simulink model "Firsts_OPTION"  (R2023a)
settings: Solver=FixedStepAuto  StartTime=0.0  StopTime=inf  FixedStep=0.01  RelTol=1e-3  EnableMultiTasking=on
libraries: arduinolib x35, dspfdesign x10, slpidlib x5
settings Model: ExtModeTrigDuration=2  Creator=PHUC  LastModifiedBy=PHUC
settings SolverCC: AutoInsertRateTranBlk=on
settings OptimizationCC: EnhancedBackFolding=on  PassReuseOutputArgsAs=Individual arguments  ZeroExternalMemoryAtStartup=off  ZeroInternalMemoryAtStartup=off  MaxStackSize=64  OptimizeBlockOrder=speed  DifferentSizesBufferReuse=on  OptimizationCustomize=off  EfficientTunableParamExpr=on
settings DebuggingCC: ParameterTunabilityLossMsg=error
settings HardwareCC: ProdBitPerInt=16  ProdBitPerPointer=16  ProdBitPerSizeT=16  ProdBitPerPtrDiffT=16  ProdLargestAtomicFloat=None  ProdWordSize=8  ProdHWDeviceType=Atmel->AVR
settings SFSimCC: MATLABDynamicMemAlloc=off
settings RTWCC: Description=Embedded Coder  SystemTargetFile=ert.tlc  HardwareBoard=Arduino Mega 2560  TemplateMakefile=ert_default_tmf  Toolchain=Arduino AVR  BuildConfiguration=Faster Runs
settings CodeAppCC: ForceParamTrailComments=on  IgnoreCustomStorageClasses=off  OperatorAnnotations=on  SimulinkDataObjDesc=on  SFDataObjDesc=on  InsertBlockDesc=on
settings ERTTargetCC: SupportContinuousTime=on  SupportVariableSizeSignals=on  ExtModeTransport=3  ExtModeStaticAlloc=on  ExtModeAutomaticAllocSize=off  ExtModeStaticAllocSize=2048  ExtModeMexFile=ext_xcp  ExtModeIntrfLevel=Level2 - Open

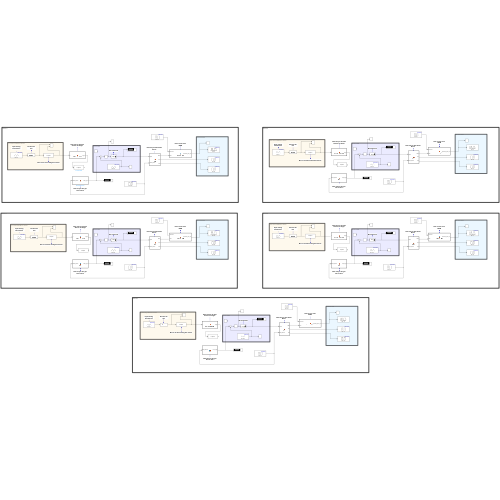
[thumbnail: Simulink's stored preview of the top-level diagram]
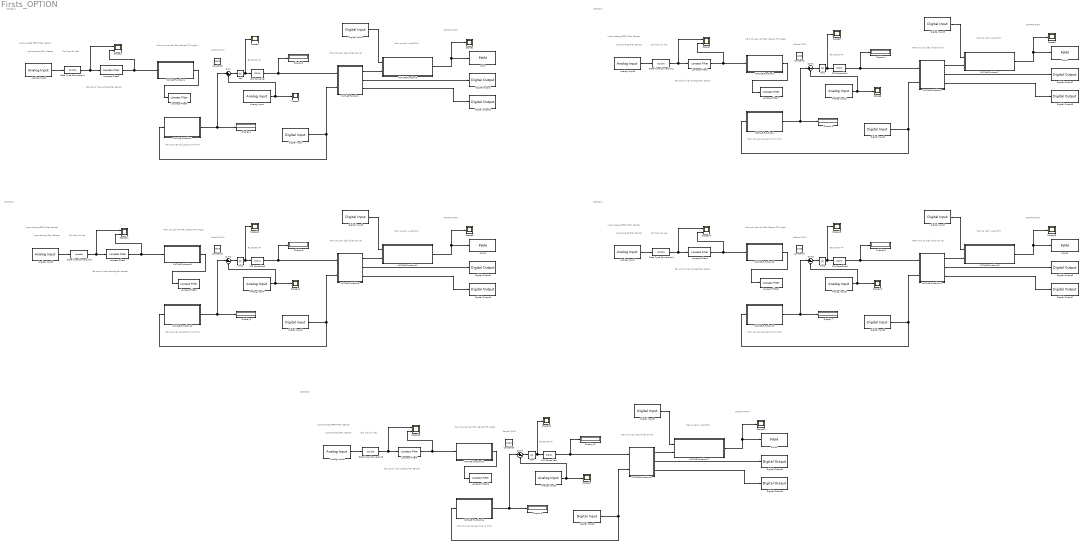
== system Firsts_OPTION ==
  note: MOTOR 1
  note: OUTPUT PWM
  note: Bo Control PI
  note: Control PWM
  note: Ham chuyen doi Flex Sensor TO Angle
  note: Doi kieu du lieu
  note: Bo Loc tin hieu analog flex sensor
  note: Input Analog FROM Flex Sensor
  note: Input analog Flex Sensor
  note: Ham chuyen dieu khien Driver
  note: Ham chuyen doi goc Hut va Thoi
  note: Ham ra lenh xuat PWM
  note: Ham ra lenh xuat PWM
  note: Doi kieu du lieu
  note: Ham chuyen doi Flex Sensor TO Angle
  note: Input analog Flex Sensor
  note: OUTPUT PWM
  note: Input Analog FROM Flex Sensor
  note: Control PWM
  note: Bo Control PI
  note: Bo Loc tin hieu analog flex sensor
  note: Ham chuyen dieu khien Driver
  note: Ham chuyen doi goc Hut va Thoi
  note: Ham ra lenh xuat PWM
  note: Control PWM
  note: Ham chuyen doi goc Hut va Thoi
  note: Input Analog FROM Flex Sensor
  note: Bo Control PI
  note: Ham chuyen dieu khien Driver
  note: Input analog Flex Sensor
  note: Bo Loc tin hieu analog flex sensor
  note: Ham chuyen doi Flex Sensor TO Angle
  note: Doi kieu du lieu
  note: OUTPUT PWM
  note: Control PWM
  note: Doi kieu du lieu
  note: Ham chuyen dieu khien Driver
  note: Ham chuyen doi Flex Sensor TO Angle
  note: OUTPUT PWM
  note: Bo Loc tin hieu analog flex sensor
  note: Bo Control PI
  note: Ham ra lenh xuat PWM
  note: Input Analog FROM Flex Sensor
  note: Input analog Flex Sensor
  note: Ham chuyen doi goc Hut va Thoi
  note: Input analog Flex Sensor
  note: Ham chuyen doi Flex Sensor TO Angle
  note: Bo Loc tin hieu analog flex sensor
  note: OUTPUT PWM
  note: Input Analog FROM Flex Sensor
  note: Ham chuyen doi goc Hut va Thoi
  note: Ham chuyen dieu khien Driver
  note: Bo Control PI
  note: Doi kieu du lieu
  note: Ham ra lenh xuat PWM
  note: Control PWM
  note: MOTOR 2
  note: MOTOR 5
  note: MOTOR 4
  note: MOTOR 3
  Abs{,1..4} (5 alike) : Abs  SaturateOnIntegerOverflow=off
  Analog Input : arduinolib/Analog Input  pinNumber=8  ReadResultsOnly=off  ConversionTriggerSource=Software  ExternalTriggerType=uint32( 0 )  OutputDataType=uint16  EnableConversionCompleteNotify=off  EnableOuputStatus=off  SampleTime=-1  blockPlatform=arduino
  Analog Input1 : arduinolib/Analog Input  pinNumber=0  ReadResultsOnly=off  ConversionTriggerSource=Software  ExternalTriggerType=uint32( 0 )  OutputDataType=uint16  EnableConversionCompleteNotify=off  EnableOuputStatus=off  SampleTime=-1  blockPlatform=arduino
  Analog Input2 : arduinolib/Analog Input  pinNumber=9  ReadResultsOnly=off  ConversionTriggerSource=Software  ExternalTriggerType=uint32( 0 )  OutputDataType=uint16  EnableConversionCompleteNotify=off  EnableOuputStatus=off  SampleTime=-1  blockPlatform=arduino
  Analog Input3 : arduinolib/Analog Input  pinNumber=1  ReadResultsOnly=off  ConversionTriggerSource=Software  ExternalTriggerType=uint32( 0 )  OutputDataType=uint16  EnableConversionCompleteNotify=off  EnableOuputStatus=off  SampleTime=-1  blockPlatform=arduino
  Analog Input4 : arduinolib/Analog Input  pinNumber=10  ReadResultsOnly=off  ConversionTriggerSource=Software  ExternalTriggerType=uint32( 0 )  OutputDataType=uint16  EnableConversionCompleteNotify=off  EnableOuputStatus=off  SampleTime=-1  blockPlatform=arduino
  Analog Input5 : arduinolib/Analog Input  pinNumber=2  ReadResultsOnly=off  ConversionTriggerSource=Software  ExternalTriggerType=uint32( 0 )  OutputDataType=uint16  EnableConversionCompleteNotify=off  EnableOuputStatus=off  SampleTime=-1  blockPlatform=arduino
  Analog Input6 : arduinolib/Analog Input  pinNumber=11  ReadResultsOnly=off  ConversionTriggerSource=Software  ExternalTriggerType=uint32( 0 )  OutputDataType=uint16  EnableConversionCompleteNotify=off  EnableOuputStatus=off  SampleTime=-1  blockPlatform=arduino
  Analog Input7 : arduinolib/Analog Input  pinNumber=3  ReadResultsOnly=off  ConversionTriggerSource=Software  ExternalTriggerType=uint32( 0 )  OutputDataType=uint16  EnableConversionCompleteNotify=off  EnableOuputStatus=off  SampleTime=-1  blockPlatform=arduino
  Analog Input8 : arduinolib/Analog Input  pinNumber=12  ReadResultsOnly=off  ConversionTriggerSource=Software  ExternalTriggerType=uint32( 0 )  OutputDataType=uint16  EnableConversionCompleteNotify=off  EnableOuputStatus=off  SampleTime=-1  blockPlatform=arduino
  Analog Input9 : arduinolib/Analog Input  pinNumber=4  ReadResultsOnly=off  ConversionTriggerSource=Software  ExternalTriggerType=uint32( 0 )  OutputDataType=uint16  EnableConversionCompleteNotify=off  EnableOuputStatus=off  SampleTime=-1  blockPlatform=arduino
  Constant{1..5} (5 alike) : Constant  Value=1023
  Data Type Conversion{1..5} (5 alike) : DataTypeConversion  OutDataTypeStr=double  SaturateOnIntegerOverflow=off  RndMeth=Floor
  Digital Input : arduinolib/Digital Input  pinNumber=34  mode=Default  Direction=input  SampleTime=0.1  blockPlatform=arduino
  Digital Input1 : arduinolib/Digital Input  pinNumber=24  mode=Default  Direction=input  SampleTime=0.1  blockPlatform=arduino
  Digital Input2 : arduinolib/Digital Input  pinNumber=36  mode=Default  Direction=input  SampleTime=0.1  blockPlatform=arduino
  Digital Input3 : arduinolib/Digital Input  pinNumber=26  mode=Default  Direction=input  SampleTime=0.1  blockPlatform=arduino
  Digital Input4 : arduinolib/Digital Input  pinNumber=38  mode=Default  Direction=input  SampleTime=0.1  blockPlatform=arduino
  Digital Input5 : arduinolib/Digital Input  pinNumber=28  mode=Default  Direction=input  SampleTime=0.1  blockPlatform=arduino
  Digital Input6 : arduinolib/Digital Input  pinNumber=40  mode=Default  Direction=input  SampleTime=0.1  blockPlatform=arduino
  Digital Input7 : arduinolib/Digital Input  pinNumber=30  mode=Default  Direction=input  SampleTime=0.1  blockPlatform=arduino
  Digital Input8 : arduinolib/Digital Input  pinNumber=42  mode=Default  Direction=input  SampleTime=0.1  blockPlatform=arduino
  Digital Input9 : arduinolib/Digital Input  pinNumber=32  mode=Default  Direction=input  SampleTime=0.1  blockPlatform=arduino
  Digital Output : arduinolib/Digital Output  pinNumber=25  Direction=output  blockPlatform=arduino
  Digital Output1 : arduinolib/Digital Output  pinNumber=27  Direction=output  blockPlatform=arduino
  Digital Output2 : arduinolib/Digital Output  pinNumber=29  Direction=output  blockPlatform=arduino
  Digital Output3 : arduinolib/Digital Output  pinNumber=31  Direction=output  blockPlatform=arduino
  Digital Output4 : arduinolib/Digital Output  pinNumber=33  Direction=output  blockPlatform=arduino
  Digital Output5 : arduinolib/Digital Output  pinNumber=35  Direction=output  blockPlatform=arduino
  Digital Output6 : arduinolib/Digital Output  pinNumber=37  Direction=output  blockPlatform=arduino
  Digital Output7 : arduinolib/Digital Output  pinNumber=39  Direction=output  blockPlatform=arduino
  Digital Output8 : arduinolib/Digital Output  pinNumber=41  Direction=output  blockPlatform=arduino
  Digital Output9 : arduinolib/Digital Output  pinNumber=43  Direction=output  blockPlatform=arduino
  Display{1..10} (10 alike) : Display
  Lowpass Filter{1..5} (5 alike) : dspfdesign/Lowpass Filter  FilterType=FIR  DesignForMinimumOrder=off  FilterOrder=200  PassbandFrequency=0.1e3  StopbandFrequency=12e3  PassbandRipple=0.01  StopbandAttenuation=50  SampleRateMode=Specify on dialog  SampleRate=44100  SimulateUsing=Interpreted execution  roundingMode=Floor  coeffsDataTypeStr=fixdt(1,16)
  Lowpass Filter{6..10} (5 alike) : dspfdesign/Lowpass Filter  FilterType=FIR  DesignForMinimumOrder=off  FilterOrder=30  PassbandFrequency=0.01e2  StopbandFrequency=12e3  PassbandRipple=0.001  StopbandAttenuation=50  SampleRateMode=Specify on dialog  SampleRate=44100  SimulateUsing=Interpreted execution  roundingMode=Floor  coeffsDataTypeStr=fixdt(1,16)
  MATLAB Function : MATLAB Function  TreatAsAtomicUnit=on
  MATLAB Function1 : MATLAB Function  TreatAsAtomicUnit=on
  MATLAB Function10 : MATLAB Function  TreatAsAtomicUnit=on
  MATLAB Function11 : MATLAB Function  TreatAsAtomicUnit=on
  MATLAB Function12 : MATLAB Function  TreatAsAtomicUnit=on
  MATLAB Function13 : MATLAB Function  TreatAsAtomicUnit=on
  MATLAB Function14 : MATLAB Function  TreatAsAtomicUnit=on
  MATLAB Function15 : MATLAB Function  TreatAsAtomicUnit=on
  MATLAB Function16 : MATLAB Function  TreatAsAtomicUnit=on
  MATLAB Function17 : MATLAB Function  TreatAsAtomicUnit=on
  MATLAB Function18 : MATLAB Function  TreatAsAtomicUnit=on
  MATLAB Function19 : MATLAB Function  TreatAsAtomicUnit=on
  MATLAB Function2 : MATLAB Function  TreatAsAtomicUnit=on
  MATLAB Function3 : MATLAB Function  TreatAsAtomicUnit=on
  MATLAB Function4 : MATLAB Function  TreatAsAtomicUnit=on
  MATLAB Function5 : MATLAB Function  TreatAsAtomicUnit=on
  MATLAB Function6 : MATLAB Function  TreatAsAtomicUnit=on
  MATLAB Function7 : MATLAB Function  TreatAsAtomicUnit=on
  MATLAB Function8 : MATLAB Function  TreatAsAtomicUnit=on
  MATLAB Function9 : MATLAB Function  TreatAsAtomicUnit=on
  PID Controller{,1..4} (5 alike) : slpidlib/PID Controller  Controller=PID  Form=Parallel  TimeDomain=Discrete-time  UseExternalTs=off  SampleTime=0.01  IntegratorMethod=Forward Euler  FilterMethod=Forward Euler  ControllerParametersSource=internal  P=7  I=0.8  UseKiTs=off  D=0  N=100  UseFilter=on  TunerSelectOption=Transfer Function Based (PID Tuner App)  InitialConditionSource=internal  InitialConditionForIntegrator=0  InitialConditionForFilter=0  DifferentiatorICPrevScaledInput=0  ExternalReset=none  TrackingMode=off  Kt=1  LimitOutput=on  SatLimitsSource=internal  UpperSaturationLimit=160  LowerSaturationLimit=0  LinearizeAsGain=on  AntiWindupMode=back-calculation  Kb=1  LimitIntegrator=off  UpperIntegratorSaturationLimit=inf  LowerIntegratorSaturationLimit=-inf  POutMin=[]  POutMax=[]  IOutMin=[]  IOutMax=[]  DOutMin=[]  DOutMax=[]  NOutMin=[]  NOutMax=[]  SumOutMin=[]  SumOutMax=[]  SaturationOutMin=[]  SaturationOutMax=[]  PParamMin=[]  PParamMax=[]  IParamMin=[]  IParamMax=[]  DParamMin=[]  DParamMax=[]  NParamMin=[]  NParamMax=[]  KbParamMin=[]  KbParamMax=[]  KtParamMin=[]  KtParamMax=[]  KbOutMin=[]  KbOutMax=[]  KtOutMin=[]  KtOutMax=[]  IntegratorOutMin=[]  IntegratorOutMax=[]  FilterOutMin=[]  FilterOutMax=[]  SumI1OutMin=[]  SumI1OutMax=[]  SumI2OutMin=[]  SumI2OutMax=[]  SumI3OutMin=[]  SumI3OutMax=[]  SumI4OutMin=[]  SumI4OutMax=[]  SumDOutMin=[]  SumDOutMax=[]  DifferentiatorOutMin=[]  DifferentiatorOutMax=[]  FilterDiffOutCoefMin=[]  FilterDiffOutCoefMax=[]  ReciprocalOutMin=[]  ReciprocalOutMax=[]  SumDenOutMin=[]  SumDenOutMax=[]  SumNumOutMin=[]  SumNumOutMax=[]  DivideOutMin=[]  DivideOutMax=[]  UdiffTsProdOutMin=[]  UdiffTsProdOutMax=[]  NTsProdOutMin=[]  NTsProdOutMax=[]  UintegralTsProdOutMin=[]  UintegralTsProdOutMax=[]  UngainTsProdOutMin=[]  UngainTsProdOutMax=[]  ClampingZeroOutDataTypeStr=Inherit: Inherit via back propagation  ClampingZeroOutMin=[]  ClampingZeroOutMax=[]  FilterDenConstantOutDataTypeStr=Inherit: Inherit via back propagation  FilterDenConstantOutMin=[]  FilterDenConstantOutMax=[]  PCopyOutDataTypeStr=Inherit: Inherit via back propagation  PCopyOutMin=[]  PCopyOutMax=[]  NCopyOutDataTypeStr=Inherit: Inherit via back propagation  NCopyOutMin=[]  NCopyOutMax=[]  IntegratorContinuousStateAttributes=''  IntegratorStateMustResolveToSignalObject=off  IntegratorRTWStateStorageClass=Auto  FilterContinuousStateAttributes=''  FilterStateMustResolveToSignalObject=off  FilterRTWStateStorageClass=Auto  ParallelPVariant=InternalParameters  IdealPVariant=Disabled  IVariant=InternalParameters  DVariant=InternalParameters  IntegratorVariant=Discrete  SatVariant=Enabled  AWVariant=BackCalculation  PCopyVariant=Disabled  TRVariant=Disabled  FdbkBlocksVariant=Forward  IdealPFdbkVariant=Disabled  SatFdbkVariant=Disabled  DerivativeFilterVariant=ForwardEulerFilter  NVariant=InternalParameters  NCopyVariant=Disabled  FilterICVariant=InternalICsFilter  IntegratorICVariant=InternalICs  ExternalResetVariant=Disabled  TRSumVariant=Passthrough  SumFdbkVariant=Disabled  SumVariant=Sum_PID  TsampFilterVariant=InternalTs  TsampNgainVariant=Passthrough  TsampIntegralVariant=Disabled_SignalSpec  ExternalSaturationOutDataTypeStr=Inherit: Same as second input
  PWM : arduinolib/PWM  pinNumber=8  frequencyType=Default  desiredFrequency=490.2  achievableFrequency=490.2
  PWM1 : arduinolib/PWM  pinNumber=9  frequencyType=Default  desiredFrequency=490.2  achievableFrequency=490.2
  PWM2 : arduinolib/PWM  pinNumber=10  frequencyType=Default  desiredFrequency=490.2  achievableFrequency=490.2
  PWM3 : arduinolib/PWM  pinNumber=11  frequencyType=Default  desiredFrequency=490.2  achievableFrequency=490.2
  PWM4 : arduinolib/PWM  pinNumber=12  frequencyType=Default  desiredFrequency=490.2  achievableFrequency=490.2
  Scope{1..2,4..6,8..10,12..13,15..17,19..20} (15 alike) : Scope
  Scope{3,7,11,14,18} (5 alike) : Scope  NumInputPorts=2
  Sum{,1..4} (5 alike) : Sum  Inputs=|+-
  wires:
  MATLAB Function/2(IN1) -> Digital Output/1
  MATLAB Function/3(IN2) -> Digital Output1/1
  PID Controller/1 -> Display2/1, MATLAB Function/1(speed)
  Digital Input/1 -> MATLAB Function/2(Blend_Stretch), MATLAB Function2/1(Blend_Stretch)
  Analog Input/1 -> Scope2/1, Sum/2
  Analog Input1/1 -> Data Type Conversion1/1
  Data Type Conversion1/1 -> Lowpass Filter3/1, Scope3/1
  Lowpass Filter3/1 -> Scope3/2, MATLAB Function1/1(u)
  MATLAB Function2/1(Limit_angle) -> Sum/1, Display1/1
  Sum/1 -> Abs/1
  Abs/1 -> Scope4/1, PID Controller/1
  Digital Input1/1 -> MATLAB Function3/1(command)
  MATLAB Function/1(ENA) -> MATLAB Function3/2(pwm)
  MATLAB Function3/1(command_pwm_out) -> Scope1/1, PWM/1
  MATLAB Function4/1(ENA) -> MATLAB Function7/2(pwm)
  MATLAB Function6/1(Limit_angle) -> Sum1/1, Display3/1
  Digital Input3/1 -> MATLAB Function7/1(command)
  MATLAB Function7/1(command_pwm_out) -> Scope5/1, PWM1/1
  Digital Input2/1 -> MATLAB Function4/2(Blend_Stretch), MATLAB Function6/1(Blend_Stretch)
  Lowpass Filter1/1 -> Scope7/2, MATLAB Function5/1(u)
  Analog Input2/1 -> Scope6/1, Sum1/2
  PID Controller1/1 -> Display4/1, MATLAB Function4/1(speed)
  Sum1/1 -> Abs1/1
  Analog Input3/1 -> Data Type Conversion2/1
  MATLAB Function4/3(IN2) -> Digital Output3/1
  MATLAB Function4/2(IN1) -> Digital Output2/1
  Data Type Conversion2/1 -> Lowpass Filter1/1, Scope7/1
  Abs1/1 -> Scope8/1, PID Controller1/1
  Lowpass Filter2/1 -> Scope11/2, MATLAB Function9/1(u)
  Abs2/1 -> Scope12/1, PID Controller2/1
  MATLAB Function8/2(IN1) -> Digital Output4/1
  MATLAB Function8/3(IN2) -> Digital Output5/1
  Analog Input5/1 -> Data Type Conversion3/1
  Data Type Conversion3/1 -> Lowpass Filter2/1, Scope11/1
  Sum2/1 -> Abs2/1
  Analog Input4/1 -> Scope10/1, Sum2/2
  PID Controller2/1 -> Display6/1, MATLAB Function8/1(speed)
  MATLAB Function8/1(ENA) -> MATLAB Function11/2(pwm)
  MATLAB Function10/1(Limit_angle) -> Sum2/1, Display5/1
  Digital Input5/1 -> MATLAB Function11/1(command)
  Digital Input4/1 -> MATLAB Function8/2(Blend_Stretch), MATLAB Function10/1(Blend_Stretch)
  MATLAB Function11/1(command_pwm_out) -> Scope9/1, PWM2/1
  Sum3/1 -> Abs3/1
  Data Type Conversion4/1 -> Lowpass Filter4/1, Scope14/1
  Analog Input7/1 -> Data Type Conversion4/1
  MATLAB Function14/2(IN1) -> Digital Output6/1
  PID Controller3/1 -> Display8/1, MATLAB Function14/1(speed)
  Digital Input6/1 -> MATLAB Function14/2(Blend_Stretch), MATLAB Function12/1(Blend_Stretch)
  Digital Input7/1 -> MATLAB Function13/1(command)
  MATLAB Function12/1(Limit_angle) -> Sum3/1, Display7/1
  MATLAB Function13/1(command_pwm_out) -> Scope16/1, PWM3/1
  MATLAB Function14/1(ENA) -> MATLAB Function13/2(pwm)
  Abs3/1 -> Scope15/1, PID Controller3/1
  MATLAB Function14/3(IN2) -> Digital Output7/1
  Analog Input6/1 -> Scope13/1, Sum3/2
  Lowpass Filter4/1 -> Scope14/2, MATLAB Function15/1(u)
  Analog Input9/1 -> Data Type Conversion5/1
  PID Controller4/1 -> Display10/1, MATLAB Function18/1(speed)
  Digital Input9/1 -> MATLAB Function17/1(command)
  MATLAB Function17/1(command_pwm_out) -> Scope20/1, PWM4/1
  MATLAB Function18/1(ENA) -> MATLAB Function17/2(pwm)
  MATLAB Function16/1(Limit_angle) -> Sum4/1, Display9/1
  Digital Input8/1 -> MATLAB Function18/2(Blend_Stretch), MATLAB Function16/1(Blend_Stretch)
  Abs4/1 -> Scope19/1, PID Controller4/1
  MATLAB Function18/2(IN1) -> Digital Output8/1
  Analog Input8/1 -> Scope17/1, Sum4/2
  Data Type Conversion5/1 -> Lowpass Filter5/1, Scope18/1
  MATLAB Function18/3(IN2) -> Digital Output9/1
  Lowpass Filter5/1 -> Scope18/2, MATLAB Function19/1(u)
  Sum4/1 -> Abs4/1
  MATLAB Function1/1(Angle) -> Lowpass Filter6/1
  MATLAB Function5/1(Angle) -> Lowpass Filter7/1
  MATLAB Function15/1(Angle) -> Lowpass Filter8/1
  MATLAB Function9/1(Angle) -> Lowpass Filter9/1
  MATLAB Function19/1(Angle) -> Lowpass Filter10/1

== matlab function Firsts_OPTION/MATLAB Function9 ==
  data: u input; Angle output
function Angle  = convert_flex_sensor(u)

VCC = 4.98;
R_DIV = 47500.0;
STRAIGHT_RESISTANCE = 24000.0;
BEND_RESISTANCE = 30000.0;


flexV = u * VCC / 1023.0;
flexR = R_DIV * (VCC / flexV - 1.0);

Angle = (((flexR - STRAIGHT_RESISTANCE)/(BEND_RESISTANCE - STRAIGHT_RESISTANCE))*90.0);

== matlab function Firsts_OPTION/MATLAB Function12 ==
  data: Blend_Stretch input; Limit_angle output
function Limit_angle = fcn(Blend_Stretch)

if Blend_Stretch == 0
    Limit_angle = 1023;
else
    Limit_angle = -3;
end

== matlab function Firsts_OPTION/MATLAB Function1 ==
  data: u input; Angle output
function Angle  = convert_flex_sensor(u)

VCC = 4.98;
R_DIV = 47500.0;
STRAIGHT_RESISTANCE = 24000.0;
BEND_RESISTANCE = 30000.0;


flexV = u * VCC / 1023.0;
flexR = R_DIV * (VCC / flexV - 1.0);

Angle = (((flexR - STRAIGHT_RESISTANCE)/(BEND_RESISTANCE - STRAIGHT_RESISTANCE))*90.0);

== matlab function Firsts_OPTION/MATLAB Function13 ==
  data: command input; pwm input; command_pwm_out output
function command_pwm_out  = Command_PWM(command, pwm)

if command == 1
    command_pwm_out = pwm;
else
    command_pwm_out = 0;
end

== matlab function Firsts_OPTION/MATLAB Function14 ==
  data: speed input; ENA output; Blend_Stretch input; IN1 output; IN2 output
function [ENA, IN1, IN2] = Driver(speed, Blend_Stretch)

ENA = abs(speed);

if Blend_Stretch == 1
    IN1 = 1;
    IN2 = 0;
else
    IN1 = 0;
    IN2 = 1;
end

== matlab function Firsts_OPTION/MATLAB Function15 ==
  data: u input; Angle output
function Angle  = convert_flex_sensor(u)

VCC = 4.98;
R_DIV = 47500.0;
STRAIGHT_RESISTANCE = 24000.0;
BEND_RESISTANCE = 30000.0;


flexV = u * VCC / 1023.0;
flexR = R_DIV * (VCC / flexV - 1.0);

Angle = (((flexR - STRAIGHT_RESISTANCE)/(BEND_RESISTANCE - STRAIGHT_RESISTANCE))*90.0);

== matlab function Firsts_OPTION/MATLAB Function16 ==
  data: Blend_Stretch input; Limit_angle output
function Limit_angle = fcn(Blend_Stretch)

if Blend_Stretch == 0
    Limit_angle = 1023;
else
    Limit_angle = -3;
end

== matlab function Firsts_OPTION/MATLAB Function17 ==
  data: command input; pwm input; command_pwm_out output
function command_pwm_out  = Command_PWM(command, pwm)

if command == 1
    command_pwm_out = pwm;
else
    command_pwm_out = 0;
end

== matlab function Firsts_OPTION/MATLAB Function18 ==
  data: speed input; ENA output; Blend_Stretch input; IN1 output; IN2 output
function [ENA, IN1, IN2] = Driver(speed, Blend_Stretch)

ENA = abs(speed);

if Blend_Stretch == 1
    IN1 = 1;
    IN2 = 0;
else
    IN1 = 0;
    IN2 = 1;
end

== matlab function Firsts_OPTION/MATLAB Function19 ==
  data: u input; Angle output
function Angle  = convert_flex_sensor(u)

VCC = 4.98;
R_DIV = 47500.0;
STRAIGHT_RESISTANCE = 24000.0;
BEND_RESISTANCE = 30000.0;


flexV = u * VCC / 1023.0;
flexR = R_DIV * (VCC / flexV - 1.0);

Angle = (((flexR - STRAIGHT_RESISTANCE)/(BEND_RESISTANCE - STRAIGHT_RESISTANCE))*90.0);

== matlab function Firsts_OPTION/MATLAB Function ==
  data: speed input; ENA output; Blend_Stretch input; IN1 output; IN2 output
function [ENA, IN1, IN2] = Driver(speed, Blend_Stretch)

ENA = abs(speed);

if Blend_Stretch == 1
    IN1 = 1;
    IN2 = 0;
else
    IN1 = 0;
    IN2 = 1;
end

== matlab function Firsts_OPTION/MATLAB Function2 ==
  data: Blend_Stretch input; Limit_angle output
function Limit_angle = fcn(Blend_Stretch)

if Blend_Stretch == 0
    Limit_angle = 1023;
else
    Limit_angle = -3;
end

== matlab function Firsts_OPTION/MATLAB Function3 ==
  data: command input; pwm input; command_pwm_out output
function command_pwm_out  = Command_PWM(command, pwm)

if command == 1
    command_pwm_out = pwm;
else
    command_pwm_out = 0;
end

== matlab function Firsts_OPTION/MATLAB Function4 ==
  data: speed input; ENA output; Blend_Stretch input; IN1 output; IN2 output
function [ENA, IN1, IN2] = Driver(speed, Blend_Stretch)

ENA = abs(speed);

if Blend_Stretch == 1
    IN1 = 1;
    IN2 = 0;
else
    IN1 = 0;
    IN2 = 1;
end

== matlab function Firsts_OPTION/MATLAB Function5 ==
  data: u input; Angle output
function Angle  = convert_flex_sensor(u)

VCC = 4.98;
R_DIV = 47500.0;
STRAIGHT_RESISTANCE = 24000.0;
BEND_RESISTANCE = 30000.0;


flexV = u * VCC / 1023.0;
flexR = R_DIV * (VCC / flexV - 1.0);

Angle = (((flexR - STRAIGHT_RESISTANCE)/(BEND_RESISTANCE - STRAIGHT_RESISTANCE))*90.0);

== matlab function Firsts_OPTION/MATLAB Function6 ==
  data: Blend_Stretch input; Limit_angle output
function Limit_angle = fcn(Blend_Stretch)

if Blend_Stretch == 0
    Limit_angle = 1023;
else
    Limit_angle = -3;
end

== matlab function Firsts_OPTION/MATLAB Function7 ==
  data: command input; pwm input; command_pwm_out output
function command_pwm_out  = Command_PWM(command, pwm)

if command == 1
    command_pwm_out = pwm;
else
    command_pwm_out = 0;
end

== matlab function Firsts_OPTION/MATLAB Function10 ==
  data: Blend_Stretch input; Limit_angle output
function Limit_angle = fcn(Blend_Stretch)

if Blend_Stretch == 0
    Limit_angle = 1023;
else
    Limit_angle = -3;
end

== matlab function Firsts_OPTION/MATLAB Function11 ==
  data: command input; pwm input; command_pwm_out output
function command_pwm_out  = Command_PWM(command, pwm)

if command == 1
    command_pwm_out = pwm;
else
    command_pwm_out = 0;
end

== matlab function Firsts_OPTION/MATLAB Function8 ==
  data: speed input; ENA output; Blend_Stretch input; IN1 output; IN2 output
function [ENA, IN1, IN2] = Driver(speed, Blend_Stretch)

ENA = abs(speed);

if Blend_Stretch == 1
    IN1 = 1;
    IN2 = 0;
else
    IN1 = 0;
    IN2 = 1;
end
